simulink subsystem "Subsystem"  (R2025b)
settings: Solver=VariableStepAuto  StartTime=0.0  StopTime=10.0  RelTol=1e-3
model mask{Waterlevel_1=275, Height=1, Max_cap_1=300, Diameter=24.5, K=7.77*1e-5, A=0.0117, B=0.1252, Duration_S1=10, Flowrate_S1=1, BurstStart=1, BurstFlow=1, BurstDur=1, RainSwitch_S1=on, Waterlevel_2=150, Height_2=1, Max_cap_2=300, Diameter_2=24.5, K_2=7.77*1e-5, A_2=0.0117, B_2=0.1252, Duration_S2=10, Flowrate_S2=1, BurstStart_2=1, BurstFlow_2=1, BurstDur_2=1, RainSwitch_S2=on, DelayLength=10}
  mask prompts: Waterlevel_1 "Initial water level:"; Max_cap_1 "Max capacity:"; A "Valve coeff A:"; Duration_S1 "Duration (sec):"; Flowrate_S1 "Flowrate (liters/min):"; BurstStart "Burst start:"; BurstFlow "Burst flow:"; BurstDur "Burst duration:"; RainSwitch_S1 "Set rain on/off"; Waterlevel_2 "Initial water level:"; Height_2 "Height:"; Max_cap_2 "Max capacity:"; Diameter_2 "Diameter:"; K_2 "K:"; A_2 "Valve coeff A:"; B_2 "B:"; Duration_S2 "Duration (sec):"; Flowrate_S2 "Flowrate (liters/min):"; BurstStart_2 "Burst start:"; BurstFlow_2 "Burst flow:"; BurstDur_2 "Burst duration:"; RainSwitch_S2 "Set rain on/off"; DelayLength "Transport delay(sec):"
settings Model: Creator=klump  LastModifiedBy=klump

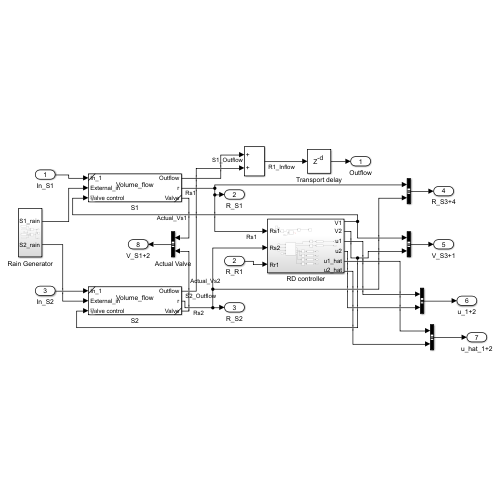
[thumbnail: Simulink's stored preview of the top-level diagram]
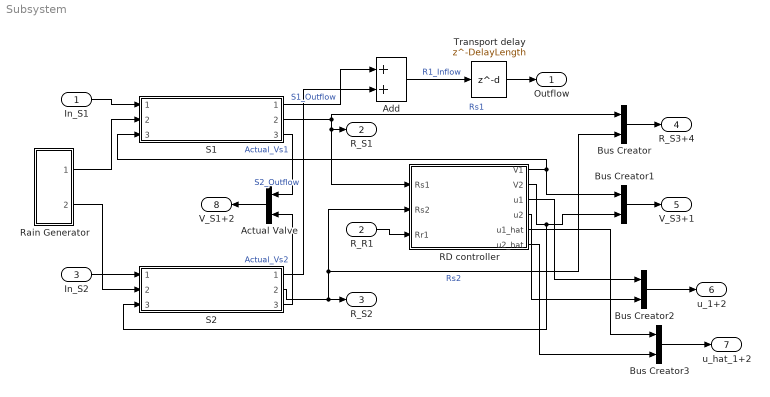
== system Subsystem ==
  In_S1 : Inport
  R_R1 : Inport  Port=2
  In_S2 : Inport  Port=3
  Actual Valve : BusCreator  Inputs=2
  Add : Sum
  Bus Creator{,1..3} (4 alike) : BusCreator  Inputs=2
  RD controller : Subsystem
  Rain Generator : Subsystem
  S1 : Subsystem  ReferencedSubsystem=Volume_flow  InitialCondition=Waterlevel_1  Max_cap=Max_cap_1  Diameter=Diameter  K=K  Height=Height  A=A  B=B
  S2 : Subsystem  ReferencedSubsystem=Volume_flow  InitialCondition=Waterlevel_2  Max_cap=Max_cap_2  Diameter=Diameter_2  K=K_2  Height=Height_2  A=A_2  B=B_2
  Transport delay : Delay  DelayLength=DelayLength  InputProcessing=Columns as channels (frame based)
  Outflow : Outport
  R_S1 : Outport  Port=2
  R_S2 : Outport  Port=3
  R_S3+4 : Outport  Port=4
  V_S3+1 : Outport  Port=5
  u_1+2 : Outport  Port=6
  u_hat_1+2 : Outport  Port=7
  V_S1+2 : Outport  Port=8
  wires:
  In_S2/1 -> S2/1
  R_R1/1 -> RD controller/3(Rr1)
  S2/2 -> R_S2/1, RD controller/2(Rs2), Bus Creator/2  "Rs2"
  RD controller/2(V2) -> S2/3, Bus Creator1/2
  Bus Creator/1 -> R_S3+4/1
  Bus Creator1/1 -> V_S3+1/1
  Add/1 -> Transport delay/1  "R1_Inflow"
  Transport delay/1 -> Outflow/1
  S2/1 -> Add/2  "S2_Outflow"
  RD controller/3(u1) -> Bus Creator2/1
  RD controller/4(u2) -> Bus Creator2/2
  Bus Creator2/1 -> u_1+2/1
  Bus Creator3/1 -> u_hat_1+2/1
  RD controller/5(u1_hat) -> Bus Creator3/1
  RD controller/6(u2_hat) -> Bus Creator3/2
  S1/2 -> Bus Creator/1, R_S1/1, RD controller/1(Rs1)  "Rs1"
  S1/1 -> Add/1  "S1_Outflow"
  RD controller/1(V1) -> S1/3, Bus Creator1/1
  Rain Generator/1(S1_rain) -> S1/2
  In_S1/1 -> S1/1
  Rain Generator/2(S2_rain) -> S2/2
  Actual Valve/1 -> V_S1+2/1
  S1/3 -> Actual Valve/1  "Actual_Vs1"
  S2/3 -> Actual Valve/2  "Actual_Vs2"

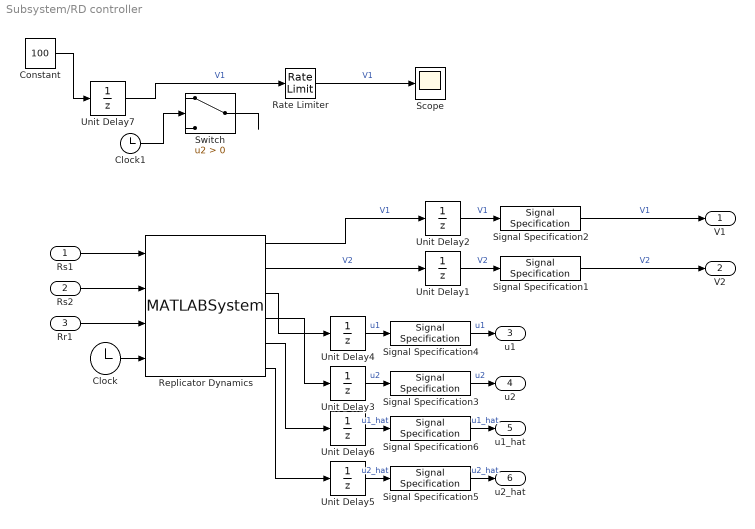
== system Subsystem/RD controller ==
  Rs1 : Inport
  Rs2 : Inport  Port=2
  Rr1 : Inport  Port=3
  Clock : Clock
  Clock1 : Clock
  Constant : Constant  Value=100
  Rate Limiter : RateLimiter  RisingSlewLimit=11.11  FallingSlewLimit=-11.11  SampleTimeMode=inherited
  Replicator Dynamics : MATLABSystem  System=RD_controller  SimulateUsing=Interpreted execution
      mask Type: RD_controller
  Scope : Scope
      settings: ActiveDisplayYMinimum=-12.499999999999996  ActiveDisplayYMaximum=112.5  DataLoggingVariableName=ScopeData18
  Signal Specification{1..6} (6 alike) : SignalSpecification  Dimensions=1
  Switch : Switch  Criteria=u2 > Threshold  SaturateOnIntegerOverflow=off  InputSameDT=off
  Unit Delay{1..7} (7 alike) : UnitDelay  SampleTime=-1  HasFrameUpgradeWarning=on
  V1 : Outport
  V2 : Outport  Port=2
  u1 : Outport  Port=3
  u2 : Outport  Port=4
  u1_hat : Outport  Port=5
  u2_hat : Outport  Port=6
  wires:
  Unit Delay7/1 -> Rate Limiter/1  "V1"
  Rate Limiter/1 -> Scope/1  "V1"
  Switch/1 -> ?
  Clock1/1 -> Switch/2
  Constant/1 -> Unit Delay7/1
  Replicator Dynamics/6 -> Unit Delay5/1
  Replicator Dynamics/5 -> Unit Delay6/1
  Unit Delay5/1 -> Signal Specification5/1  "u2_hat"
  Signal Specification6/1 -> u1_hat/1  "u1_hat"
  Signal Specification5/1 -> u2_hat/1  "u2_hat"
  Unit Delay6/1 -> Signal Specification6/1  "u1_hat"
  Replicator Dynamics/4 -> Unit Delay3/1
  Replicator Dynamics/3 -> Unit Delay4/1
  Unit Delay3/1 -> Signal Specification3/1  "u2"
  Unit Delay4/1 -> Signal Specification4/1  "u1"
  Signal Specification3/1 -> u2/1  "u2"
  Signal Specification4/1 -> u1/1  "u1"
  Rr1/1 -> Replicator Dynamics/3
  Rs2/1 -> Replicator Dynamics/2
  Rs1/1 -> Replicator Dynamics/1
  Clock/1 -> Replicator Dynamics/4
  Unit Delay2/1 -> Signal Specification2/1  "V1"
  Signal Specification2/1 -> V1/1  "V1"
  Unit Delay1/1 -> Signal Specification1/1  "V2"
  Signal Specification1/1 -> V2/1  "V2"
  Replicator Dynamics/2 -> Unit Delay1/1  "V2"
  Replicator Dynamics/1 -> Unit Delay2/1  "V1"

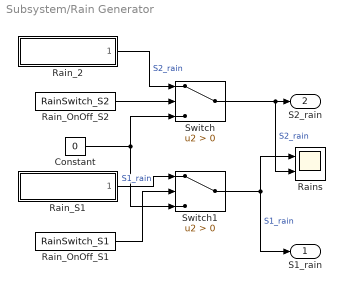
== system Subsystem/Rain Generator ==
  Constant : Constant  Value=0
  Rain_2 : Subsystem  ReferencedSubsystem=Rain  Duration=Duration_S2  Flowrate=Flowrate_S2  BurstStart=BurstStart_2  BurstFlow=BurstFlow_2  BurstDur=BurstDur_2
  Rain_OnOff_S1 : Constant  Value=RainSwitch_S1
  Rain_OnOff_S2 : Constant  Value=RainSwitch_S2
  Rain_S1 : Subsystem  ReferencedSubsystem=Rain  Duration=Duration_S1  Flowrate=Flowrate_S1  BurstStart=BurstStart  BurstFlow=BurstFlow  BurstDur=BurstDur
  Rains : Scope  NumInputPorts=2
      settings: ActiveDisplayYMinimum=-1  ActiveDisplayYMaximum=1  DataLoggingVariableName=ScopeData2
  Switch : Switch  Criteria=u2 > Threshold  SaturateOnIntegerOverflow=off  InputSameDT=off
  Switch1 : Switch  Criteria=u2 > Threshold  SaturateOnIntegerOverflow=off  InputSameDT=off
  S1_rain : Outport
  S2_rain : Outport  Port=2
  wires:
  Rain_OnOff_S1/1 -> Switch1/2
  Rain_2/1 -> Switch/1  "S2_rain"
  Rain_S1/1 -> Switch1/1  "S1_rain"
  Constant/1 -> Switch1/3, Switch/3
  Switch1/1 -> S1_rain/1, Rains/1  "S1_rain"
  Rain_OnOff_S2/1 -> Switch/2
  Switch/1 -> S2_rain/1, Rains/2  "S2_rain"
